simulink model "lab02_2"  (Simulink 10.3)
settings: Solver=VariableStepAuto  StartTime=0.0  StopTime=10  RelTol=1e-3
values from neighbouring files (symbols this model uses):
  c_1 = 0.2254    [lab02.mat]    (also in lab03.mat; lab04.mat; lab05.mat; lab06.mat)
  c_r = 0.0144    [lab02.mat]    (also in lab03.mat; lab04.mat; lab05.mat; lab06.mat)
  g = 9.8    [lab02.mat]    (also in lab03.mat; lab04.mat; lab05.mat; lab06.mat)
  Ja = 0.06904489    [lab02.mat]    (also in lab03.mat; lab04.mat; lab05.mat = 0.06191089; lab06.mat = 0.06932089)
  Jb = 0.04317025    [lab02.mat]    (also in lab03.mat; lab04.mat; lab05.mat = 0.03603625; lab06.mat = 0.04344625)
  k_a = 2546    [lab02.mat]    (also in lab03.mat; lab04.mat; lab05.mat; lab06.mat)
  k_f = 0.0013    [lab02.mat]    (also in lab03.mat; lab04.mat; lab05.mat; lab06.mat)
  k_s = 32    [lab02.mat]    (also in lab03.mat; lab04.mat; lab05.mat; lab06.mat)
  k_x = 50200    [lab02.mat]    (also in lab03.mat; lab04.mat; lab05.mat; lab06.mat)
  l_0 = 0.33    [lab02.mat]    (also in lab03.mat; lab04.mat; lab05.mat; lab06.mat)
  l_c = -0.0458067226891    [lab03.mat]    (also in lab04.mat; lab05.mat = -0.0295602240896; lab06.mat = -0.0463669467787; lab07.mat = -0.0295602240896)
  m_1 = 0.2376    [lab02.mat]    (also in lab03.mat; lab04.mat; lab05.mat; lab06.mat)
  m_2 = 1.785    [lab02.mat]    (also in lab03.mat; lab04.mat; lab05.mat; lab06.mat)
settings Model: Creator=kisdev  LastModifiedBy=kisdev
settings SolverCC: AlgebraicLoopSolver=Auto
settings DataIOCC: SaveFormat=Dataset  SignalLoggingSaveFormat=Dataset  ReturnWorkspaceOutputs=on
settings OptimizationCC: ExpressionDepthLimit=128  LifeSpan=auto
settings DebuggingCC: UnderspecifiedInitializationDetection=Simplified  MergeDetectMultiDrivingBlocksExec=error  FcnCallInpInsideContextMsg=error  StateNameClashWarn=none  SFUnexpectedBacktrackingDiag=error  SFNoUnconditionalDefaultTransitionDiag=error  SFExecutionAtInitializationDiag=warning  SFMachineParentedDataDiag=error  ArithmeticOperatorsInVariantConditions=error
settings HardwareCC: ProdBitPerPointer=64  ProdBitPerSizeT=64  ProdBitPerPtrDiffT=64  ProdLargestAtomicFloat=Float  ProdIntDivRoundTo=Zero  ProdEndianess=LittleEndian  ProdWordSize=64  ProdHWDeviceType=Intel->x86-64 (Windows64)
settings ModelReferenceCC: PropagateSignalLabelsOutOfModel=on
settings SFSimCC: SimUseLocalCustomCode=on  CustomCodeUndefinedFunction=FilterOut
settings RTWCC: RTWUseLocalCustomCode=on
settings CodeAppCC: StateflowObjectComments=off
settings GRTTargetCC: TargetLangStandard=C99 (ISO)  CombineOutputUpdateFcns=on  GRTInterface=off
settings ConfigComp: CovMetricSettings=dwe  CovSaveCumulativeToWorkspaceVar=off  CovSaveSingleToWorkspaceVar=off  CovExternalEMLEnable=on

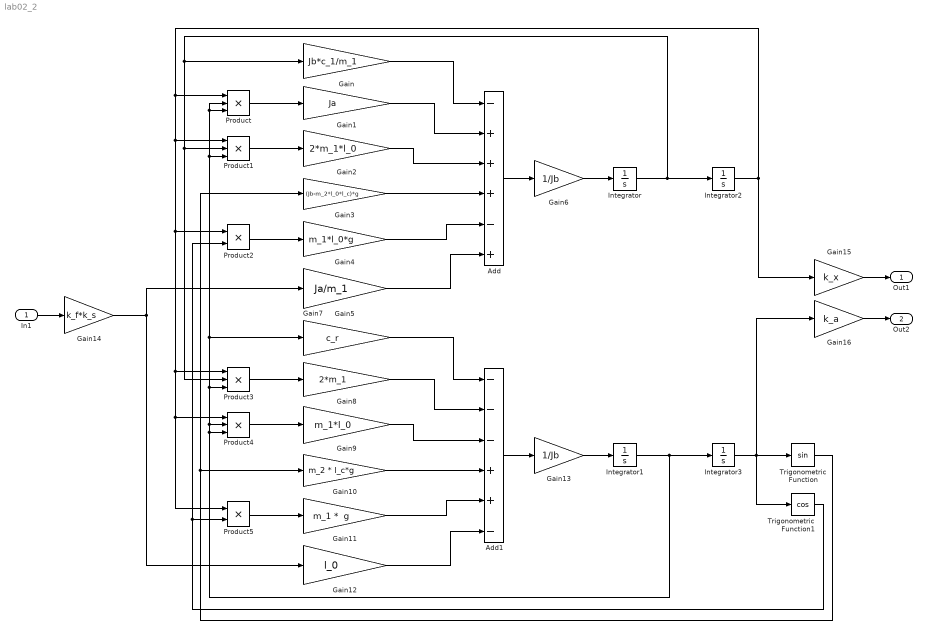
== system lab02_2 ==
  In1 : Inport
  Add : Sum  Inputs=-+++-+
  Add1 : Sum  Inputs=---++-
  Gain : Gain  Gain=Jb*c_1/m_1
  Gain1 : Gain  Gain=Ja
  Gain10 : Gain  Gain=m_2 * l_c*g
  Gain11 : Gain  Gain="m_1 *  g"
  Gain12 : Gain  Gain=l_0
  Gain13 : Gain  Gain=1/Jb
  Gain14 : Gain  Gain=k_f*k_s
  Gain15 : Gain  Gain=k_x
  Gain16 : Gain  Gain=k_a
  Gain2 : Gain  Gain=2*m_1*l_0
  Gain3 : Gain  Gain=(Jb-m_2*l_0*l_c)*g
  Gain4 : Gain  Gain=m_1*l_0*g
  Gain5 : Gain  Gain=Ja/m_1
  Gain6 : Gain  Gain=1/Jb
  Gain7 : Gain  Gain=c_r
  Gain8 : Gain  Gain=2*m_1
  Gain9 : Gain  Gain=m_1*l_0
  Integrator{,1..3} (4 alike) : Integrator
  Product{,1,3..4} (4 alike) : Product  Inputs=3
  Product2 : Product
  Product5 : Product
  Trigonometric Function : Trigonometry
  Trigonometric Function1 : Trigonometry  Operator=cos
  Out1 : Outport  SignalName=x
  Out2 : Outport  Port=2  SignalName=theta
  wires:
  Gain5/1 -> Add/6
  Gain4/1 -> Add/5
  Gain3/1 -> Add/4
  Gain2/1 -> Add/3
  Gain1/1 -> Add/2
  Gain/1 -> Add/1
  Gain6/1 -> Integrator/1
  Add/1 -> Gain6/1
  Gain11/1 -> Add1/5
  Gain9/1 -> Add1/3
  Gain13/1 -> Integrator1/1
  Gain8/1 -> Add1/2
  Gain7/1 -> Add1/1
  Gain12/1 -> Add1/6
  Add1/1 -> Gain13/1
  Gain10/1 -> Add1/4
  Integrator1/1 -> Product4/3, Product4/2, Product3/3, Gain7/1, Product1/3, Product/3, Product/2, Integrator3/1
  Integrator/1 -> Gain/1, Product3/2, Product1/2, Integrator2/1
  Integrator3/1 -> Gain16/1, Trigonometric Function1/1, Trigonometric Function/1
  Product2/1 -> Gain4/1
  Product1/1 -> Gain2/1
  Product/1 -> Gain1/1
  Product3/1 -> Gain8/1
  Product4/1 -> Gain9/1
  Product5/1 -> Gain11/1
  Integrator2/1 -> Gain15/1, Product5/1, Product4/1, Product3/1, Product2/1, Product1/1, Product/1
  Trigonometric Function/1 -> Gain10/1, Gain3/1
  Trigonometric Function1/1 -> Product5/2, Product2/2
  In1/1 -> Gain14/1
  Gain14/1 -> Gain12/1, Gain5/1
  Gain15/1 -> Out1/1
  Gain16/1 -> Out2/1
